simulink model "test"  (R2014a)
settings: Solver=FixedStepDiscrete  StartTime=0.0  StopTime=inf  FixedStep=Tsim  RelTol=1e-3
undefined symbols (not defined in the file or in its folder): Tsim
libraries: geometry_msgs x2, active_estimation_msgs x2, rt_sync x1
settings Model: SimulationMode=rapid-accelerator  ExtModeTrigDuration=100  Creator=rspica  LastModifiedBy=rspica
settings DataIOCC: SaveFinalState=on  SaveFormat=StructureWithTime  SaveOutput=off  SaveState=on  StateSaveName=tmp_raccel_xout  SignalLoggingName=tmp_raccel_logsout
settings OptimizationCC: ExpressionDepthLimit=2147483647  EfficientMapNaN2IntZero=off
settings DebuggingCC: UnderspecifiedInitializationDetection=Classic  StateNameClashWarn=warning
settings HardwareCC: TargetBitPerLong=64  TargetBitPerPointer=64  TargetLongLongMode=on  TargetIntDivRoundTo=Zero  TargetEndianess=LittleEndian  TargetWordSize=64  TargetHWDeviceType=MATLAB Host  ProdEqTarget=off
settings RTWCC: SystemTargetFile=raccel.tlc  TemplateMakefile=raccel_default_tmf  RTWVerbose=off  ProcessScript=raccel_make_rtw_hook  RTWUseSimCustomCode=on
settings CodeAppCC: GenerateComments=off  MaxIdLength=128  MangleLength=10  SimulinkBlockComments=off
settings RaccelTargetCC: ERTMultiwordTypeDef=System defined  ERTMultiwordLength=256  GeneratePreprocessorConditionals=Disable all  ERTFirstTimeCompliant=off  MultiInstanceERTCode=off  EnableShiftOperators=on  ExtModeMexArgs='', 0, 54400  ENABLE_SLEXEC_SSBRIDGE=0  RTWCAPIParams=off

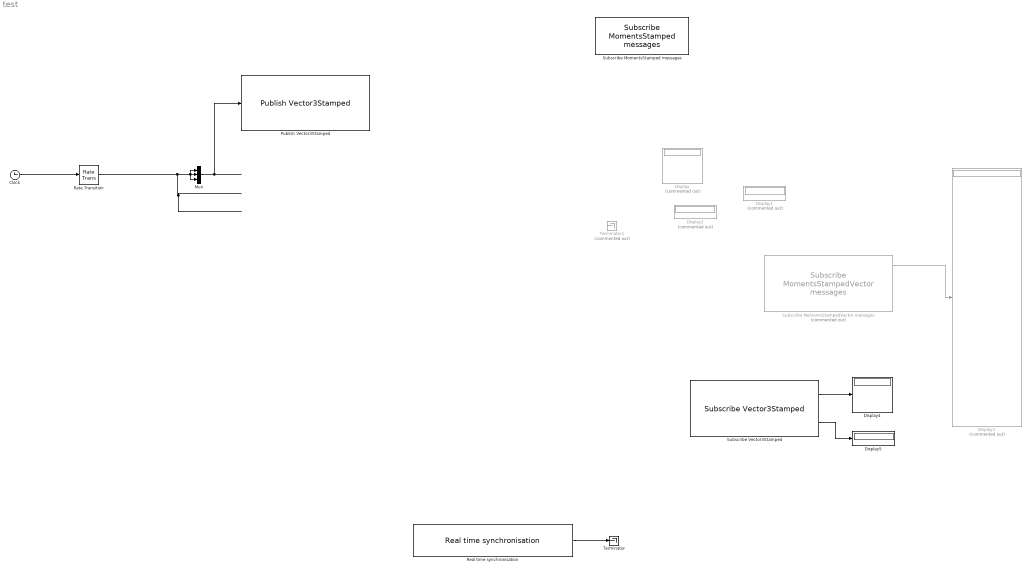
== system test ==
  Clock : Clock
  Display{,1..3} (4 alike) : Display  Commented=on
  Display4 : Display
  Display5 : Display
  Mux : Mux  Inputs=3
  Publish Vector3Stamped : geometry_msgs/Publish Vector3Stamped  stepTime=Tsim  topic_prefix='/Vector3_'  list_of_robot_ids=char([0])  topic_postfix=''
  Rate Transition : RateTransition
  Real time synchronisation : rt_sync/Real time synchronisation  stepTime=Tsim  minShownDelay=0.5  ShowEveryNumCycles=1/Tsim  slowDownFactor=1
  Subscribe MomentsStamped messages : active_estimation_msgs/Subscribe MomentsStamped messages  stepTime=Tsim  topic_prefix='Moments_'  list_of_ids=char([0])  topic_postfix=''
  Subscribe MomentsStampedVector messages : active_estimation_msgs/Subscribe MomentsStampedVector messages  Commented=on  stepTime=Tsim  topic_prefix='/ros_image_'  list_of_ids=char([0])  topic_postfix='/Feature'  max_size=char(100)
  Subscribe Vector3Stamped : geometry_msgs/Subscribe Vector3Stamped  stepTime=Tsim  topic_prefix='/Vector3_'  list_of_robot_ids=char([0])  topic_postfix=''
  Terminator : Terminator
  Terminator1 : Terminator  Commented=on
  wires:
  Clock/1 -> Rate Transition/1
  Mux/1 -> Publish Vector3Stamped/1
  Real time synchronisation/1 -> Terminator/1
  Rate Transition/1 -> Mux/3, Mux/2, Mux/1
  ? -> Display/1
  ? -> Display1/1
  ? -> Display2/1
  ? -> Terminator1/1
  Subscribe MomentsStampedVector messages/1 -> Display3/1
  Subscribe Vector3Stamped/1 -> Display4/1
  Subscribe Vector3Stamped/2 -> Display5/1
